simulink model "s_qube2_bal_PID"  (R2022b)
settings: Solver=ode1  StartTime=0.0  StopTime=5  FixedStep=Ts  MaxStep=0.02  MinStep=0.001  RelTol=1e-3  EnableMultiTasking=on
values from neighbouring files (symbols this model uses):
  bp = 5e-5    (= 5e-05)    [LQR_SetParams.m]    (also in PID_SetParams.m; qube2_rotpen_param.m)
  br = 1e-3    (= 0.001)    [LQR_SetParams.m]    (also in PID_SetParams.m; qube2_rotpen_param.m)
  g = 9.81    [LQR_SetParams.m]    (also in PID_SetParams.m; qube2_rotpen_param.m)
  I_D = SL.I_D    [PID_MainScript.m]
  I_I = SL.I_I    [PID_MainScript.m]
  I_P = SL.I_P    [PID_MainScript.m]
  ic_alpha0 = pi*170/180    (= 2.96705972839)    [LQR_SetParams.m]    (also in PID_SetParams.m)
  Jp = mp*Lp^2/3    (= 0.000133128)    [LQR_SetParams.m]    (also in PID_SetParams.m; qube2_rotpen_param.m)
  Jr = mr*r^2/3    (= 0.000228791666667)    [LQR_SetParams.m]    (also in PID_SetParams.m; qube2_rotpen_param.m)
  km = 0.042    [LQR_SetParams.m]    (also in PID_SetParams.m; inverted_pendulum_matlab.m; qube2_rotpen_param.m)
  kt = 0.042    [LQR_SetParams.m]    (also in PID_SetParams.m; inverted_pendulum_matlab.m; qube2_rotpen_param.m)
  l = -1    [LQR_SetParams.m]    (also in PID_SetParams.m = 0.0645; inverted_pendulum_matlab.m; qube2_rotpen_param.m = 0.0645)
  mp = 0.024    [LQR_SetParams.m]    (also in PID_SetParams.m; qube2_rotpen_param.m)
  O_D = SL.O_D    [PID_MainScript.m]
  O_I = SL.O_I    [PID_MainScript.m]
  O_P = SL.O_P    [PID_MainScript.m]
  r = 0.085    [LQR_SetParams.m]    (also in PID_SetParams.m; qube2_rotpen_param.m)
  Rm = 9.7    [LQR_SetParams.m]    (also in PID_SetParams.m; qube2_rotpen_param.m)
  theta_max = pi/3    (= 1.0471975512)    [LQR_SetParams.m]    (also in PID_SetParams.m)
  Vmax = 5    [LQR_SetParams.m]    (also in PID_SetParams.m)
libraries: slpidlib x2, simulink_extras x2
settings Model: ExtModeTrigDuration=5000  Creator=MLevis  LastModifiedBy=maxlg
settings SolverCC: InitialStep=Ts  AlgebraicLoopSolver=TrustRegion
settings DebuggingCC: UnderspecifiedInitializationDetection=Classic  MergeDetectMultiDrivingBlocksExec=none  UnconnectedInputMsg=warning  UnconnectedOutputMsg=warning  UnconnectedLineMsg=warning  SFMachineParentedDataDiag=warning
settings ModelReferenceCC: EnableRefExpFcnMdlSchedulingChecks=on  PropagateSignalLabelsOutOfModel=off
settings SFSimCC: CustomCodeUndefinedFunction=UseInterfaceOnly
settings RTWCC: DLArmComputeVersion=19.05

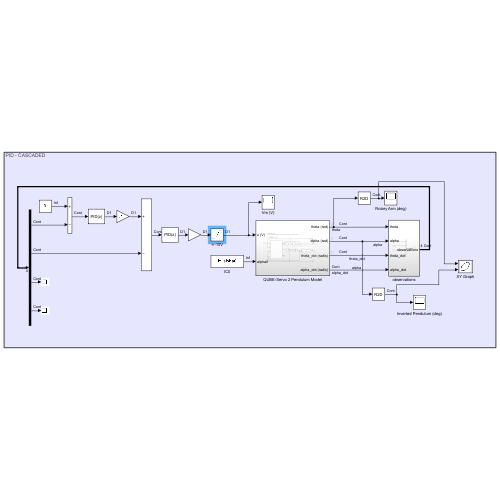
[thumbnail: Simulink's stored preview of the top-level diagram]
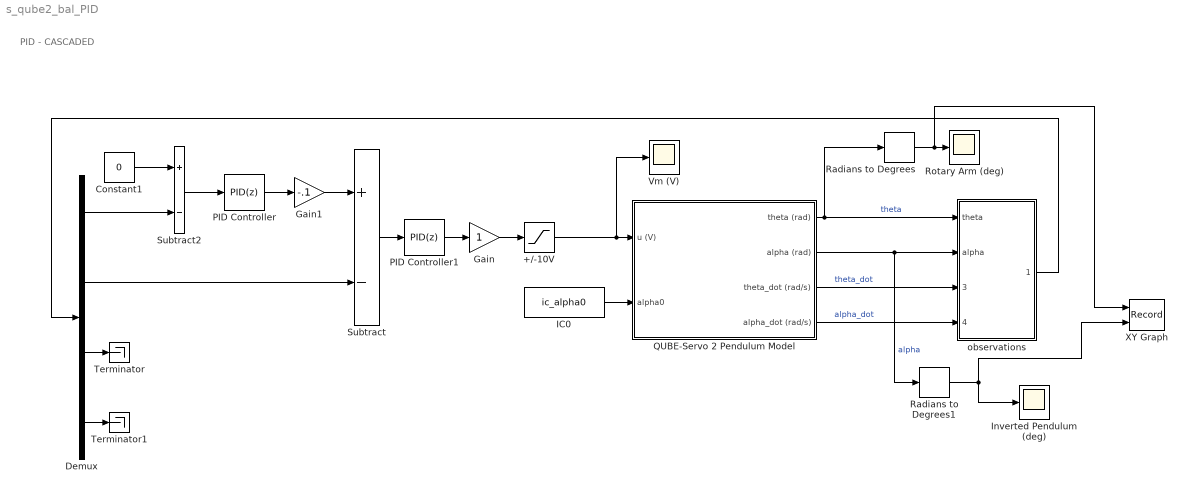
== system s_qube2_bal_PID ==
  note: PID - CASCADED
  +/-10V : Saturate  UpperLimit=Vmax  LowerLimit=-Vmax  OutDataTypeStr=Inherit: Inherit via back propagation
  Constant1 : Constant  Value=0
  Demux : Demux
  Gain : Gain
  Gain1 : Gain  Gain=-.1
  IC0 : Constant  Value=ic_alpha0
  Inverted Pendulum (deg) : Scope
  PID Controller : slpidlib/PID Controller  Controller=PID  Form=Parallel  TimeDomain=Discrete-time  UseExternalTs=off  SampleTime=-1  IntegratorMethod=Forward Euler  FilterMethod=Forward Euler  ControllerParametersSource=internal  P=O_P  I=O_I  UseKiTs=off  D=O_D  N=100  UseFilter=on  TunerSelectOption=Transfer Function Based (PID Tuner App)  InitialConditionSource=internal  InitialConditionForIntegrator=0  InitialConditionForFilter=0  DifferentiatorICPrevScaledInput=0  ExternalReset=none  TrackingMode=off  Kt=1  LimitOutput=off  SatLimitsSource=internal  UpperSaturationLimit=inf  LowerSaturationLimit=-inf  LinearizeAsGain=on  AntiWindupMode=none  Kb=1  LimitIntegrator=off  UpperIntegratorSaturationLimit=inf  LowerIntegratorSaturationLimit=-inf  POutMin=[]  POutMax=[]  IOutMin=[]  IOutMax=[]  DOutMin=[]  DOutMax=[]  NOutMin=[]  NOutMax=[]  SumOutMin=[]  SumOutMax=[]  SaturationOutMin=[]  SaturationOutMax=[]  PParamMin=[]  PParamMax=[]  IParamMin=[]  IParamMax=[]  DParamMin=[]  DParamMax=[]  NParamMin=[]  NParamMax=[]  KbParamMin=[]  KbParamMax=[]  KtParamMin=[]  KtParamMax=[]  KbOutMin=[]  KbOutMax=[]  KtOutMin=[]  KtOutMax=[]  IntegratorOutMin=[]  IntegratorOutMax=[]  FilterOutMin=[]  FilterOutMax=[]  SumI1OutMin=[]  SumI1OutMax=[]  SumI2OutMin=[]  SumI2OutMax=[]  SumI3OutMin=[]  SumI3OutMax=[]  SumI4OutMin=[]  SumI4OutMax=[]  SumDOutMin=[]  SumDOutMax=[]  DifferentiatorOutMin=[]  DifferentiatorOutMax=[]  FilterDiffOutCoefMin=[]  FilterDiffOutCoefMax=[]  ReciprocalOutMin=[]  ReciprocalOutMax=[]  SumDenOutMin=[]  SumDenOutMax=[]  SumNumOutMin=[]  SumNumOutMax=[]  DivideOutMin=[]  DivideOutMax=[]  UdiffTsProdOutMin=[]  UdiffTsProdOutMax=[]  NTsProdOutMin=[]  NTsProdOutMax=[]  UintegralTsProdOutMin=[]  UintegralTsProdOutMax=[]  UngainTsProdOutMin=[]  UngainTsProdOutMax=[]  ClampingZeroOutDataTypeStr=Inherit: Inherit via back propagation  ClampingZeroOutMin=[]  ClampingZeroOutMax=[]  FilterDenConstantOutDataTypeStr=Inherit: Inherit via back propagation  FilterDenConstantOutMin=[]  FilterDenConstantOutMax=[]  PCopyOutDataTypeStr=Inherit: Inherit via back propagation  PCopyOutMin=[]  PCopyOutMax=[]  NCopyOutDataTypeStr=Inherit: Inherit via back propagation  NCopyOutMin=[]  NCopyOutMax=[]  IntegratorContinuousStateAttributes=''  IntegratorStateMustResolveToSignalObject=off  IntegratorRTWStateStorageClass=Auto  FilterContinuousStateAttributes=''  FilterStateMustResolveToSignalObject=off  FilterRTWStateStorageClass=Auto  ParallelPVariant=InternalParameters  IdealPVariant=Disabled  IVariant=InternalParameters  DVariant=InternalParameters  IntegratorVariant=Discrete  SatVariant=Disabled  AWVariant=Passthrough  PCopyVariant=Disabled  TRVariant=Disabled  FdbkBlocksVariant=Forward  IdealPFdbkVariant=Disabled  SatFdbkVariant=Disabled  DerivativeFilterVariant=ForwardEulerFilter  NVariant=InternalParameters  NCopyVariant=Disabled  FilterICVariant=InternalICsFilter  IntegratorICVariant=InternalICs  ExternalResetVariant=Disabled  TRSumVariant=Passthrough  SumFdbkVariant=Disabled  SumVariant=Sum_PID  TsampFilterVariant=InternalTs  TsampNgainVariant=Passthrough  TsampIntegralVariant=Passthrough  ExternalSaturationOutDataTypeStr=Inherit: Same as second input
  PID Controller1 : slpidlib/PID Controller  Controller=PID  Form=Parallel  TimeDomain=Discrete-time  UseExternalTs=off  SampleTime=-1  IntegratorMethod=Forward Euler  FilterMethod=Forward Euler  ControllerParametersSource=internal  P=I_P  I=I_I  UseKiTs=off  D=I_D  N=100  UseFilter=on  TunerSelectOption=Transfer Function Based (PID Tuner App)  InitialConditionSource=internal  InitialConditionForIntegrator=0  InitialConditionForFilter=0  DifferentiatorICPrevScaledInput=0  ExternalReset=none  TrackingMode=off  Kt=1  LimitOutput=off  SatLimitsSource=internal  UpperSaturationLimit=inf  LowerSaturationLimit=-inf  LinearizeAsGain=on  AntiWindupMode=none  Kb=1  LimitIntegrator=off  UpperIntegratorSaturationLimit=inf  LowerIntegratorSaturationLimit=-inf  POutMin=[]  POutMax=[]  IOutMin=[]  IOutMax=[]  DOutMin=[]  DOutMax=[]  NOutMin=[]  NOutMax=[]  SumOutMin=[]  SumOutMax=[]  SaturationOutMin=[]  SaturationOutMax=[]  PParamMin=[]  PParamMax=[]  IParamMin=[]  IParamMax=[]  DParamMin=[]  DParamMax=[]  NParamMin=[]  NParamMax=[]  KbParamMin=[]  KbParamMax=[]  KtParamMin=[]  KtParamMax=[]  KbOutMin=[]  KbOutMax=[]  KtOutMin=[]  KtOutMax=[]  IntegratorOutMin=[]  IntegratorOutMax=[]  FilterOutMin=[]  FilterOutMax=[]  SumI1OutMin=[]  SumI1OutMax=[]  SumI2OutMin=[]  SumI2OutMax=[]  SumI3OutMin=[]  SumI3OutMax=[]  SumI4OutMin=[]  SumI4OutMax=[]  SumDOutMin=[]  SumDOutMax=[]  DifferentiatorOutMin=[]  DifferentiatorOutMax=[]  FilterDiffOutCoefMin=[]  FilterDiffOutCoefMax=[]  ReciprocalOutMin=[]  ReciprocalOutMax=[]  SumDenOutMin=[]  SumDenOutMax=[]  SumNumOutMin=[]  SumNumOutMax=[]  DivideOutMin=[]  DivideOutMax=[]  UdiffTsProdOutMin=[]  UdiffTsProdOutMax=[]  NTsProdOutMin=[]  NTsProdOutMax=[]  UintegralTsProdOutMin=[]  UintegralTsProdOutMax=[]  UngainTsProdOutMin=[]  UngainTsProdOutMax=[]  ClampingZeroOutDataTypeStr=Inherit: Inherit via back propagation  ClampingZeroOutMin=[]  ClampingZeroOutMax=[]  FilterDenConstantOutDataTypeStr=Inherit: Inherit via back propagation  FilterDenConstantOutMin=[]  FilterDenConstantOutMax=[]  PCopyOutDataTypeStr=Inherit: Inherit via back propagation  PCopyOutMin=[]  PCopyOutMax=[]  NCopyOutDataTypeStr=Inherit: Inherit via back propagation  NCopyOutMin=[]  NCopyOutMax=[]  IntegratorContinuousStateAttributes=''  IntegratorStateMustResolveToSignalObject=off  IntegratorRTWStateStorageClass=Auto  FilterContinuousStateAttributes=''  FilterStateMustResolveToSignalObject=off  FilterRTWStateStorageClass=Auto  ParallelPVariant=InternalParameters  IdealPVariant=Disabled  IVariant=InternalParameters  DVariant=InternalParameters  IntegratorVariant=Discrete  SatVariant=Disabled  AWVariant=Passthrough  PCopyVariant=Disabled  TRVariant=Disabled  FdbkBlocksVariant=Forward  IdealPFdbkVariant=Disabled  SatFdbkVariant=Disabled  DerivativeFilterVariant=ForwardEulerFilter  NVariant=InternalParameters  NCopyVariant=Disabled  FilterICVariant=InternalICsFilter  IntegratorICVariant=InternalICs  ExternalResetVariant=Disabled  TRSumVariant=Passthrough  SumFdbkVariant=Disabled  SumVariant=Sum_PID  TsampFilterVariant=InternalTs  TsampNgainVariant=Passthrough  TsampIntegralVariant=Passthrough  ExternalSaturationOutDataTypeStr=Inherit: Same as second input
  QUBE-Servo 2 Pendulum Model : Subsystem
  Radians to Degrees : simulink_extras/Transformations/Radians to Degrees
  Radians to Degrees1 : simulink_extras/Transformations/Radians to Degrees
  Rotary Arm (deg) : Scope
  Subtract : Sum  Inputs=+-
  Subtract2 : Sum  Inputs=+-
  Terminator : Terminator
  Terminator1 : Terminator
  Vm (V) : Scope
  XY Graph : Record  FileSettingsInternal="{\"entries\":[{\"content\":{\"excelSettings\":{\"content\":{},\"type\":\"Streamout.ExcelSettings\"}},\"type\":\"Streamout.FileSettingStorage\",\"uuid\":\"07544d70-e6c4-4c15-89dd-9ea18948ce69\"}],\"packageUris\":[\"http://schema.mathworks.com/mf0/streamout_blocks/R2020a\"],\"version\":\"1.0\"}"  Layout=[1 1]  SignalsInternal="{\"entries\":[{\"content\":{\"signals\":[{\"content\":{\"blockPath\":[\"s_qube2_bal_PID/XY Graph\"],\"channel\":[],\"dimensions\":[1],\"domain\":\"s_qube2_bal_PID/XY Graph\",\"lineColor\":\"#d95319\",\"plots\":[],\"port\":1,\"sid\":[],\"signalID\":138,\"signalName\":\"Radians\\nto Degrees\"},\"type\":\"RecordBlkView.Signal\",\"uuid\":\"8759f6a1-7ccd-4fae-b87d-f7c1b71d364f\"},{\"content\":{\"blockPath\":[\"s_qube2_bal_PID/XY Graph\"],\"channel\":[],\"dimensions\":[1],\"domain\":\"s_qube2_bal_PID/XY Graph\",\"lineColor\":\"#edb120\",\"plots\":[],\"port\":2,\"sid\":[],\"signalID\":141,\"signalName\":\"Radians\\nto Degrees1\"},\"type\":\"RecordBlkView.Signal\",\"uuid\":\"dd3c5d8c-7717-46f3-98e6-2561ad5892a2\"}]},\"type\":\"RecordBlkView.InputSignals\",\"uuid\":\"165a0881-1ccf-43a6-885d-34ed21606047\"}],\"packageUris\":[\"http://schema.mathworks.com/mf0/streamout_blocks/R2020a\"],\"version\":\"1.0\"}"  VisualizationBindings="{\"xyplotplugin\":{\"info\":[{\"series\":[],\"subplotID\":1}]}}"  CompatibilityTag=XY
  observations : Subsystem  VariantControl=sincos
  wires:
  Radians to Degrees/1 -> XY Graph/1, Rotary Arm (deg)/1
  Radians to Degrees1/1 -> XY Graph/2, Inverted Pendulum (deg)/1
  +/-10V/1 -> QUBE-Servo 2 Pendulum Model/1(u (V)), Vm (V)/1
  QUBE-Servo 2 Pendulum Model/2(alpha (rad)) -> Radians to Degrees1/1, observations/2(alpha)  "alpha"
  QUBE-Servo 2 Pendulum Model/1(theta (rad)) -> Radians to Degrees/1, observations/1(theta)  "theta"
  QUBE-Servo 2 Pendulum Model/3(theta_dot (rad/s)) -> observations/3(theta_dot)  "theta_dot"
  QUBE-Servo 2 Pendulum Model/4(alpha_dot (rad/s)) -> observations/4(alpha_dot)  "alpha_dot"
  IC0/1 -> QUBE-Servo 2 Pendulum Model/2(alpha0)
  observations/1(observations) -> Demux/1
  PID Controller/1 -> Gain1/1
  PID Controller1/1 -> Gain/1
  Gain/1 -> +/-10V/1
  Demux/1 -> Subtract2/2
  Constant1/1 -> Subtract2/1
  Subtract2/1 -> PID Controller/1
  Gain1/1 -> Subtract/1
  Demux/2 -> Subtract/2
  Subtract/1 -> PID Controller1/1
  Demux/3 -> Terminator/1
  Demux/4 -> Terminator1/1

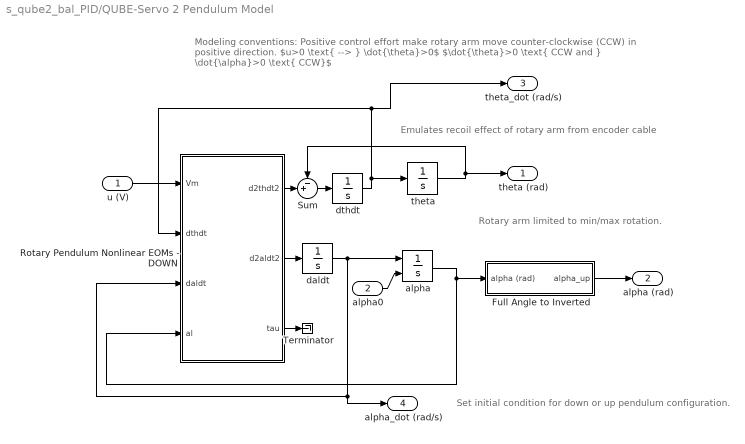
== system s_qube2_bal_PID/QUBE-Servo 2 Pendulum Model ==
  note: Rotary arm limited to min/max rotation.
  note: Modeling conventions:
      | Positive control effort make rotary arm move counter-clockwise (CCW) in positive direction.
      | $u>0 \text{ --> } \dot{\theta}>0$
      | $\dot{\theta}>0 \text{ CCW and } \dot{\alpha}>0 \text{ CCW}$
  note: Set initial condition for down or up pendulum configuration.
  note: Emulates recoil effect of rotary arm from encoder cable
  u (V) : Inport
  alpha0 : Inport  Port=2
  Full Angle to Inverted : Subsystem
  Rotary Pendulum Nonlinear EOMs - DOWN : MATLAB Function  TreatAsAtomicUnit=on
  Sum : Sum  Inputs=-+|
  Terminator : Terminator
  alpha : Integrator  InitialConditionSource=external  InitialCondition=ic_alpha0
  daldt : Integrator
  dthdt : Integrator
  theta : Integrator  LimitOutput=on  UpperSaturationLimit=theta_max  LowerSaturationLimit=-theta_max
  theta (rad) : Outport  VectorParamsAs1DForOutWhenUnconnected=off
  alpha (rad) : Outport  Port=2  VectorParamsAs1DForOutWhenUnconnected=off
  theta_dot (rad/s) : Outport  Port=3  VectorParamsAs1DForOutWhenUnconnected=off
  alpha_dot (rad/s) : Outport  Port=4  VectorParamsAs1DForOutWhenUnconnected=off
  wires:
  daldt/1 -> alpha/1, Rotary Pendulum Nonlinear EOMs - DOWN/3(daldt), alpha_dot (rad/s)/1
  alpha/1 -> Full Angle to Inverted/1(alpha (rad)), Rotary Pendulum Nonlinear EOMs - DOWN/4(al)
  Rotary Pendulum Nonlinear EOMs - DOWN/2(d2aldt2) -> daldt/1
  dthdt/1 -> theta/1, theta_dot (rad/s)/1, Rotary Pendulum Nonlinear EOMs - DOWN/2(dthdt)
  u (V)/1 -> Rotary Pendulum Nonlinear EOMs - DOWN/1(Vm)
  Rotary Pendulum Nonlinear EOMs - DOWN/3(tau) -> Terminator/1
  Full Angle to Inverted/1(alpha_up) -> alpha (rad)/1
  alpha0/1 -> alpha/2
  theta/1 -> theta (rad)/1, Sum/1
  Rotary Pendulum Nonlinear EOMs - DOWN/1(d2thdt2) -> Sum/2
  Sum/1 -> dthdt/1

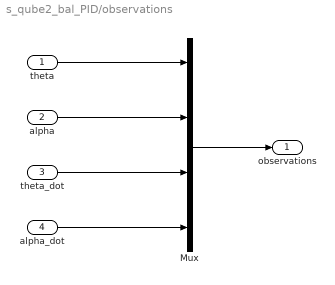
== system s_qube2_bal_PID/observations ==
  theta : Inport
  alpha : Inport  Port=2
  theta_dot : Inport  Port=3
  alpha_dot : Inport  Port=4
  Mux : Mux
  observations : Outport  VectorParamsAs1DForOutWhenUnconnected=off
  wires:
  theta/1 -> Mux/1
  alpha/1 -> Mux/2
  Mux/1 -> observations/1
  theta_dot/1 -> Mux/3
  alpha_dot/1 -> Mux/4

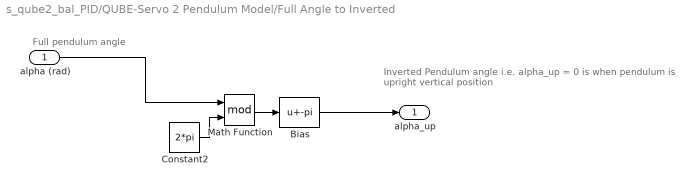
== system s_qube2_bal_PID/QUBE-Servo 2 Pendulum Model/Full Angle to Inverted ==
  note: Inverted Pendulum angle
      | i.e. alpha_up = 0 is when pendulum is upright vertical position
  note: Full pendulum angle
  alpha (rad) : Inport
  Bias : Bias  Bias=-pi  SaturateOnIntegerOverflow=off
  Constant2 : Constant  Value=2*pi
  Math Function : Math  Operator=mod  SignedPower=on
  alpha_up : Outport  VectorParamsAs1DForOutWhenUnconnected=off
  wires:
  Constant2/1 -> Math Function/2
  Bias/1 -> alpha_up/1
  alpha (rad)/1 -> Math Function/1
  Math Function/1 -> Bias/1

== matlab function s_qube2_bal_PID/QUBE-Servo 2 Pendulum Model/Rotary Pendulum Nonlinear EOMs - DOWN ==
  data: Vm input size=1; d2thdt2 output size=1; d2aldt2 output size=1; dthdt input size=1; daldt input size=1; Jp parameter; Jr parameter; l parameter; mp parameter; br parameter; bp parameter; r parameter; kt parameter; km parameter; Rm parameter; al input size=1; g parameter; tau output
function [d2thdt2,d2aldt2,tau] = pen_nonlin_eoms(Vm, dthdt, daldt, Jp, Jr, l, mp, br, bp, r, kt, km, Rm, al, g)

% Convert voltage to torque input
tau = (Vm - km*dthdt)/Rm;
tau=kt*tau;
% Denominator
Jt = Jr*Jp + Jp^2*sin(al)^2 - mp^2*r^2*l^2*cos(al)^2;
% Nonlinear equations of motion for generic rotary pendulum (i.e. furuta)
% Terms from EOM solving
term1 = tau - br*dthdt + 2*Jp*sin(al)*cos(al)*dthdt*daldt + mp*r*l*sin(al)*daldt^2;
term2 = -bp*daldt - Jp*sin(al)*cos(al)*daldt^2 - mp*g*l*sin(al);
% Torque to rotary arm position)
d2thdt2 = 1/Jt*( Jp*term1 - mp*r*l*cos(al)*term2);
% Torque to pendulum angle position
d2aldt2 = 1/Jt*(-mp*r*l*cos(al)*term1 + (Jr+Jp*sin(al)^2)*term2);
